simulink model "sim_pert_sin_ct"  (R2014b)
settings: Solver=ode45  StartTime=0.0  StopTime=25  RelTol=1e-3
values from neighbouring files (symbols this model uses):
  A = [0 -23.8095;0 0]    [Observador.m]    (also in P1.m; P1_pert.m; P1_pert_range.m; P1_pert_sin.m)
  B = [0;-23.8095]    [Observador.m]    (also in P1.m; P1_pert.m; P1_pert_range.m; P1_pert_sin.m)
  C = [1 0]    [Observador.m]    (also in P1.m; P1_pert.m = eye(2); P1_pert_range.m = eye(2); P1_pert_sin.m = eye(2))
  C_pert = eye(3)    [P1_pert.m]    (also in P1_pert_range.m = eye(5); P1_pert_sin.m = eye(4); P1_pert_sin_ct.m = eye(5); P1_pert_sin_ct_imag.m = eye(5))
  D = [0;0]    [Observador.m]    (also in P1.m; P1_pert.m; P1_pert_range.m; P1_pert_sin.m)
  gam_pert = [gam; 0]    [P1_pert.m]    (also in P1_pert_range.m = [gam; zeros(3,1)]; P1_pert_sin.m = [gam; 0; 0]; P1_pert_sin_ct.m = [gam; 0; 0; 0]; P1_pert_sin_ct_imag.m = [gam; 0; 0; 0])
  K_dis = acker(phi,gam,P_dis)    [Observador.m]    (also in P1.m; P1_pert.m; P1_pert_range.m; P1_pert_sin.m)
  L_pert = K_obs_dis_pert'    [P1_pert.m]    (also in P1_pert_range.m; P1_pert_sin.m; P1_pert_sin_ct.m; P1_pert_sin_ct_imag.m)
  phi_pert = [phi gam; 0 0 1]    [P1_pert.m]    (also in P1_pert_range.m = [phi gam*C_d [0;0]; zeros(2,2) phi_sin [0;0]; zeros(1,4) 1]; P1_pert_sin.m = [phi gam [0;0]; zeros(2) phi_sin]; P1_pert_sin_ct.m = [phi gam gam [0;0]; zeros(3,2) [1;0;0] [[0 0]; phi_sin]]; P1_pert_sin_ct_imag.m = [phi gam gam [0;0]; zeros(3,2) [1;0;0] [[0 0]; phi_sin]])
  w = 2.4*2*pi()    [P1_pert_sin.m]    (also in P1_pert_sin_ct.m = 0.5371*2*pi(); P1_pert_sin_ct_imag.m; Pert_sin.m; Pert_sin_ct.m = 0.5371*2*pi())
libraries: simulink x1
settings Model: Creator=student  LastModifiedBy=lluis
settings DataIOCC: SignalLoggingSaveFormat=ModelDataLogs
settings OptimizationCC: ExpressionDepthLimit=2147483647
settings DebuggingCC: UnderspecifiedInitializationDetection=Classic  MergeDetectMultiDrivingBlocksExec=none  FcnCallInpInsideContextMsg=EnableAllAsWarning  StateNameClashWarn=warning
settings GRTTargetCC: CombineOutputUpdateFcns=off  GRTInterface=on

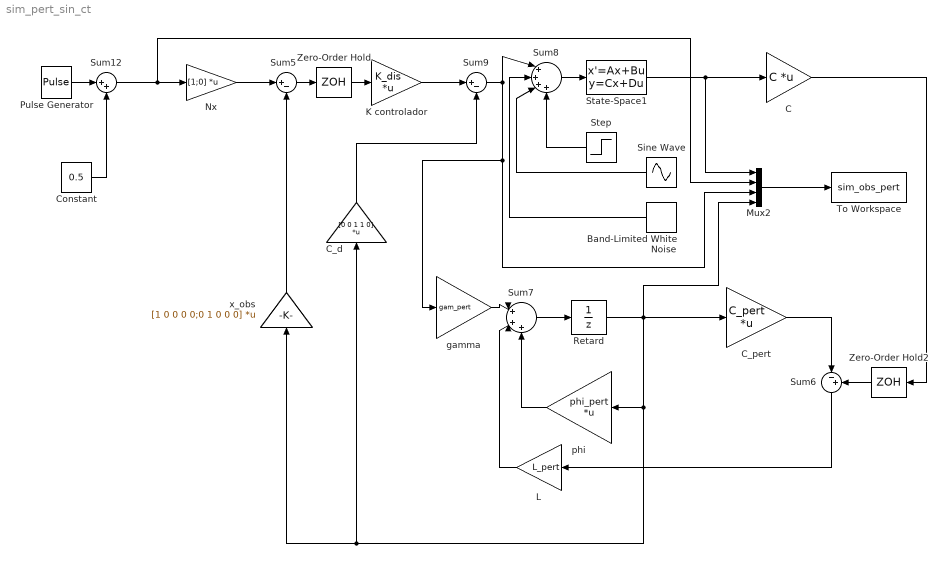
== system sim_pert_sin_ct ==
  Band-Limited White Noise : simulink/Sources/Band-Limited White Noise  Cov=[0.000001]  Ts=0.005  seed=[23341]
  C : Gain  Gain=C  Multiplication=Matrix(K*u)
  C_d : Gain  Gain=[0 0 1 1 0]  Multiplication=Matrix(K*u)
  C_pert : Gain  Gain=C_pert  Multiplication=Matrix(K*u)
  Constant : Constant  Value=0.5
  K controlador : Gain  Gain=K_dis  Multiplication=Matrix(K*u)
  L : Gain  Gain=L_pert
  Mux2 : Mux
  Nx : Gain  Gain=[1;0]  Multiplication=Matrix(K*u)
  Pulse Generator : DiscretePulseGenerator  PulseType=Time based  Amplitude=-2  Period=20  PulseWidth=50
  Retard : UnitDelay  SampleTime=-1
  Sine Wave : Sin  Amplitude=0.005  Frequency=w  SampleTime=0
  State-Space1 : StateSpace  A=A  B=B  C=eye(2)  D=D  X0=[1;1]
  Step : Step  Time=0  After=-0.05  SampleTime=0
  Sum12 : Sum  Inputs=|++
  Sum5 : Sum  Inputs=|+-
  Sum6 : Sum  Inputs=|-+
  Sum7 : Sum  Inputs=|+++
  Sum8 : Sum  Inputs=|++++
  Sum9 : Sum  Inputs=|+-
  To Workspace : ToWorkspace  VariableName=sim_obs_pert  SaveFormat=Timeseries  SampleTime=-1
  Zero-Order Hold : ZeroOrderHold  SampleTime=5E-2
  Zero-Order Hold2 : ZeroOrderHold  SampleTime=5E-2
  gamma : Gain  Gain=gam_pert
  phi : Gain  Gain=phi_pert  Multiplication=Matrix(K*u)
  x_obs : Gain  Gain=[1 0 0 0 0;0 1 0 0 0]  Multiplication=Matrix(K*u)
  wires:
  State-Space1/1 -> Mux2/1, C/1
  Sum5/1 -> Zero-Order Hold/1
  Sum12/1 -> Mux2/2, Nx/1
  Nx/1 -> Sum5/1
  Zero-Order Hold/1 -> K controlador/1
  Sum6/1 -> L/1
  gamma/1 -> Sum7/1
  L/1 -> Sum7/2
  Retard/1 -> Mux2/4, C_d/1, x_obs/1, phi/1, C_pert/1
  Sum7/1 -> Retard/1
  phi/1 -> Sum7/3
  C/1 -> Zero-Order Hold2/1
  C_pert/1 -> Sum6/1
  K controlador/1 -> Sum9/1
  Zero-Order Hold2/1 -> Sum6/2
  Sum8/1 -> State-Space1/1
  x_obs/1 -> Sum5/2
  Sum9/1 -> gamma/1, Mux2/3, Sum8/1
  C_d/1 -> Sum9/2
  Step/1 -> Sum8/4
  Sine Wave/1 -> Sum8/3
  Mux2/1 -> To Workspace/1
  Pulse Generator/1 -> Sum12/1
  Constant/1 -> Sum12/2
  Band-Limited White Noise/1 -> Sum8/2
